simulink model "Copy_of_VTOLTiltrotor"  (R2024a)
settings: configuration reference "VTOLConfiguration" (kept outside this file)
undefined symbols (not defined in the file): airspeed, Battery, BCE12, BCE_Set_init, BMS_Controller_State, C, Cell10_P, Cell11_P, Cell12_P, Cell1_N, Cell1_P, Cell2_P, Cell3_P, Cell4_P, Cell5_P, Cell6_P, Cell7_P, Cell8_P, Cell9_P, Cell_Temperatures, Cell_Voltages, Charging_State, CityMission, control, controlParams, ControlSampleTime, CriticalTiltAngle, currentFactor, CV_Gain, ddx, ddy, ddz, Device_01, DiscIntNeverNeededParam, dx, dy, dz, Earth, env, F, F28379D_ADC_MaxCount, F28379D_ADC_Vmax, FixedWingMission, flightState, Foc_Ki_IxTcpu, Foc_Ki_S, Foc_Kp_I, Foc_Kp_S, fractalcoef, FSState, FWControlParams, HoverMission, I_cc, Ia_offset, Ib_offset, iniRoll, initPitch, iniYaw, IO334, IO334_DAC_Vmax ... (+55)
libraries: slrealtimeethercatlib x109, simulink x81, fl_lib x65, slpidlib x49, mcbcontrolslib x48, nesl_utility x43, speedgoatlib_hdlCoder_IO3xx x31, canmsglib x17, slrealtimeutilitieslib x13, mcbhdlplantlib x13, speedgoatlib_IO611 x12, dspstat3 x12
(part 7 of 20)

== system Copy_of_VTOLTiltrotor/Flight Controller/Autopilot/Tilt Scheduler/Back Transition Scheduler ==
  Tilt Schedule : Inport
  FlightMode : Inport  Port=2
  States : Inport  Port=3
  Add : Sum  Inputs=+-
  Bus Selector : BusSelector  OutputSignals=Vb
  Constant1 : Constant  Value=flightState.BackTransition
  Constant6 : Constant  Value=0
  Equal1 : RelationalOperator  Operator===  OutDataTypeStr=boolean  RndMeth=Simplest  InputSameDT=off
  Saturation : Saturate  UpperLimit=pi/4  LowerLimit=-pi/4
  Selector : Selector  InputPortWidth=3  IndexOptions=Index vector (dialog)  Indices=[1]  OutputSizes=1
  Switch2 : Switch  Threshold=1  SaturateOnIntegerOverflow=off  InputSameDT=off
  Vx Controller : slpidlib/PID Controller  Controller=P  Form=Parallel  TimeDomain=Discrete-time  UseExternalTs=off  SampleTime=0.005  IntegratorMethod=Forward Euler  FilterMethod=Forward Euler  ControllerParametersSource=internal  P=controlParams.P_BACK  I=0  UseKiTs=off  D=0.0379422021775223  UseExternalDerivativeSource=off  N=1.96946409823213  UseFilter=on  TunerSelectOption=Transfer Function Based (PID Tuner App)  InitialConditionSource=internal  InitialConditionForIntegrator=0  InitialConditionForFilter=0  DifferentiatorICPrevScaledInput=0  ExternalReset=none  TrackingMode=off  Kt=1  LimitOutput=off  SatLimitsSource=internal  UpperSaturationLimit=inf  LowerSaturationLimit=-inf  LinearizeAsGain=on  AntiWindupMode=none  Kb=1  LimitIntegrator=off  UpperIntegratorSaturationLimit=inf  LowerIntegratorSaturationLimit=-inf  POutMin=[]  POutMax=[]  IOutMin=[]  IOutMax=[]  DOutMin=[]  DOutMax=[]  NOutMin=[]  NOutMax=[]  SumOutMin=[]  SumOutMax=[]  SaturationOutMin=[]  SaturationOutMax=[]  PParamMin=[]  PParamMax=[]  IParamMin=[]  IParamMax=[]  DParamMin=[]  DParamMax=[]  NParamMin=[]  NParamMax=[]  KbParamMin=[]  KbParamMax=[]  KtParamMin=[]  KtParamMax=[]  KbOutMin=[]  KbOutMax=[]  KtOutMin=[]  KtOutMax=[]  IntegratorOutMin=[]  IntegratorOutMax=[]  FilterOutMin=[]  FilterOutMax=[]  SumI1OutMin=[]  SumI1OutMax=[]  SumI2OutMin=[]  SumI2OutMax=[]  SumI3OutMin=[]  SumI3OutMax=[]  SumI4OutMin=[]  SumI4OutMax=[]  SumDOutMin=[]  SumDOutMax=[]  DifferentiatorOutMin=[]  DifferentiatorOutMax=[]  FilterDiffOutCoefMin=[]  FilterDiffOutCoefMax=[]  ReciprocalOutMin=[]  ReciprocalOutMax=[]  SumDenOutMin=[]  SumDenOutMax=[]  SumNumOutMin=[]  SumNumOutMax=[]  DivideOutMin=[]  DivideOutMax=[]  UdiffTsProdOutMin=[]  UdiffTsProdOutMax=[]  NTsProdOutMin=[]  NTsProdOutMax=[]  UintegralTsProdOutMin=[]  UintegralTsProdOutMax=[]  UngainTsProdOutMin=[]  UngainTsProdOutMax=[]  ClampingZeroOutDataTypeStr=Inherit: Inherit via back propagation  ClampingZeroOutMin=[]  ClampingZeroOutMax=[]  FilterDenConstantOutDataTypeStr=Inherit: Inherit via back propagation  FilterDenConstantOutMin=[]  FilterDenConstantOutMax=[]  PCopyOutDataTypeStr=Inherit: Inherit via back propagation  PCopyOutMin=[]  PCopyOutMax=[]  NCopyOutDataTypeStr=Inherit: Inherit via back propagation  NCopyOutMin=[]  NCopyOutMax=[]  IntegratorContinuousStateAttributes=''  IntegratorStateMustResolveToSignalObject=off  IntegratorRTWStateStorageClass=Auto  FilterContinuousStateAttributes=''  FilterStateMustResolveToSignalObject=off  FilterRTWStateStorageClass=Auto  ParallelPVariant=InternalParameters  IdealPVariant=Disabled  IVariant=Disabled  DVariant=Disabled  IntegratorVariant=Disabled  SatVariant=Disabled  AWVariant=Disabled  PCopyVariant=Disabled  TRVariant=Disabled  FdbkBlocksVariant=Forward  IdealPFdbkVariant=Disabled  SatFdbkVariant=Disabled  DerivativeFilterVariant=Disabled  NVariant=Disabled  NCopyVariant=Disabled_SignalSpec  FilterICVariant=Disabled  IntegratorICVariant=Disabled  ExternalResetVariant=Disabled  TRSumVariant=Passthrough  SumFdbkVariant=Disabled  SumVariant=Passthrough_P  TsampFilterVariant=InternalTs  TsampNgainVariant=Passthrough  TsampIntegralVariant=Disabled_SignalSpec  ExternalSaturationOutDataTypeStr=Inherit: Same as second input  DerivativeSourceVariant=Disabled
  TiltAngle : Outport
  wires:
  States/1 -> Bus Selector/1
  Add/1 -> Vx Controller/1
  Equal1/1 -> Switch2/2
  Bus Selector/1 -> Selector/1  "<Vb>"
  FlightMode/1 -> Equal1/1
  Constant1/1 -> Equal1/2
  Constant6/1 -> Add/1
  Selector/1 -> Add/2
  Vx Controller/1 -> Saturation/1
  Saturation/1 -> Switch2/1
  Tilt Schedule/1 -> Switch2/3
  Switch2/1 -> TiltAngle/1

== system Copy_of_VTOLTiltrotor/Flight Controller/Autopilot/Tilt Scheduler/Forward Transition Scheduler ==
  FlightMode : Inport
  Constant : Constant  Value=pi/2
  Constant2 : Constant  Value=0
  Constant3 : Constant  Value=CriticalTiltAngle
  Constant4 : Constant  Value=flightState.Transition
  Constant5 : Constant  Value=TiltScheduleRate
  Equal : RelationalOperator  Operator===  OutDataTypeStr=boolean  RndMeth=Simplest  InputSameDT=off
  Integrator : Integrator  ExternalReset=either  LimitOutput=on  UpperSaturationLimit=Inf  LowerSaturationLimit=0
  LessThanOrEqual : RelationalOperator  Operator=<=  OutDataTypeStr=boolean  RndMeth=Simplest  InputSameDT=off
  Switch : Switch  Criteria=u2 > Threshold  SaturateOnIntegerOverflow=off  InputSameDT=off
  Switch1 : Switch  Criteria=u2 > Threshold  SaturateOnIntegerOverflow=off  InputSameDT=off
  FlightState : Outport
  Tilt Schedule : Outport  Port=2
  tag scope: ModeFlag=global
  wires:
  FlightMode/1 -> FlightState/1, Equal/2
  [ModeFlag] -> Switch1/2, Integrator/2
  Integrator/1 -> Switch/1, LessThanOrEqual/1
  LessThanOrEqual/1 -> Switch/2
  Equal/1 -> [ModeFlag]
  Constant3/1 -> LessThanOrEqual/2
  Switch1/1 -> Integrator/1
  Constant5/1 -> Switch1/1
  Constant2/1 -> Switch1/3
  Constant4/1 -> Equal/1
  Constant/1 -> Switch/3
  Switch/1 -> Tilt Schedule/1

== system Copy_of_VTOLTiltrotor/Flight Controller/Estimator/Estimation Filter/Airspeed Filter ==
  DiffPress : Inport
  rho : Inport  Port=2
  Constant : Constant  Value=0.5
  Divide : Product  Inputs=*/
  Product : Product
  Sqrt : Sqrt
  airspeed : Outport
  wires:
  Constant/1 -> Product/2
  rho/1 -> Product/1
  Product/1 -> Divide/2
  DiffPress/1 -> Divide/1
  Divide/1 -> Sqrt/1
  Sqrt/1 -> airspeed/1

== system Copy_of_VTOLTiltrotor/Flight Controller/Estimator/Estimation Filter/LLA2Local ==
  LLA : Inport
  Constant1 : Constant  Value=0
  Demux1 : Demux  Outputs=2
  LLA to Flat Earth1 : aerolibtransform2/LLA to Flat Earth  units=Metric (MKS)  ptype=Earth (WGS84)  F=1/298.257223563  R=6378137  refPosPort=off  LL0=[0 0]  psi=0
  Xe : Outport
  wires:
  Constant1/1 -> LLA to Flat Earth1/3
  Demux1/1 -> LLA to Flat Earth1/1
  Demux1/2 -> LLA to Flat Earth1/2
  LLA to Flat Earth1/1 -> Xe/1  "Xe"
  LLA/1 -> Demux1/1

== system Copy_of_VTOLTiltrotor/Flight Controller/Ground Control Station/Get Flight Mission/noQGC ==
  note: uavPathManagerBus type
  No Mission : Constant  Value=struct('mode',0,'position',[0 0 0]','params',[0;0;0;0]);  OutDataTypeStr=Bus: doubleUavPathManager
  Variant Source : VariantSource
  Waypoints : Constant  Value=FixedWingMission  OutDataTypeStr=Bus: doubleUavPathManager  SampleTime=-1
  Waypoints1 : Constant  Value=HoverMission  OutDataTypeStr=Bus: doubleUavPathManager  SampleTime=-1
  Waypoints2 : Constant  Value=TransitionMission  OutDataTypeStr=Bus: doubleUavPathManager  SampleTime=-1
  Waypoints3 : Constant  Value=CityMission  OutDataTypeStr=Bus: doubleUavPathManager  SampleTime=-1
  Mission : Outport
  wires:
  Waypoints/1 -> Variant Source/2
  Waypoints1/1 -> Variant Source/3
  Variant Source/1 -> Mission/1
  Waypoints2/1 -> Variant Source/4
  No Mission/1 -> Variant Source/1
  Waypoints3/1 -> Variant Source/5

== system Copy_of_VTOLTiltrotor/Flight Controller/Guidance Test Bench/ControlType/Guidance Testbench ==
  Global Mission : Inport
  Aircraft States : Inport  Port=2
  Control Rate Transition : Subsystem
  Guidance Logic : Subsystem  VariantControl=guidanceType==1
  HoverCmds : Outport
  FixedWingSP : Outport  Port=2
  AACSP : Outport  Port=3
  ctrlMode : Outport  Port=4
  FlightMode : Outport  Port=5
  wires:
  Aircraft States/1 -> Guidance Logic/1(UAVState)
  Global Mission/1 -> Guidance Logic/2(GCSCommands)
  Guidance Logic/1(HoverGuidance) -> Control Rate Transition/1("1 ")
  Guidance Logic/2(FixedWingSP) -> Control Rate Transition/2(In2)
  Guidance Logic/3(AACSP) -> Control Rate Transition/3(In3)
  Guidance Logic/4(ctrlMode) -> Control Rate Transition/4(In4)
  Guidance Logic/5(FlightMode) -> Control Rate Transition/5(In5)
  Control Rate Transition/1(Out1) -> HoverCmds/1
  Control Rate Transition/2(Out2) -> FixedWingSP/1
  Control Rate Transition/3(Out3) -> AACSP/1
  Control Rate Transition/4(Out4) -> ctrlMode/1
  Control Rate Transition/5(Out5) -> FlightMode/1

== system Copy_of_VTOLTiltrotor/Flight Controller/Guidance Test Bench/ControlType/Manual Control ==
  note: Change these parameters during simulation when using manual testbench mode.
  note: Commanded Altitude (m)
  note: Commanded Y (m)
  note: Fixed Wing Aerodynamics
  note: Commanded X (m)
  note: Fixed Wing
  note: Hover
  note: Flight Mode
  note: Transition
  note: Commanded Course
  note: Commanded Altitude
  note: Commanded Airspeed (m)
  note: Back Transition
  note: Fixed Wing Commands
  note: Hover Commands
  Global Mission : Inport
  Aircraft States : Inport  Port=2
  Command Interface : Subsystem
  Slider1 : SliderBlock  LabelPosition=Hide  ScaleMax=50  TickInterval=5
  Slider2 : SliderBlock  LabelPosition=Hide  ScaleMin=-30  ScaleMax=30  TickInterval=5
  Slider3 : SliderBlock  LabelPosition=Hide  ScaleMin=-30  ScaleMax=30  TickInterval=5
  Slider4 : SliderBlock  LabelPosition=Hide  ScaleMax=3  TickInterval=1
  Slider5 : SliderBlock  LabelPosition=Hide  ScaleMin=-30  ScaleMax=30  TickInterval=5
  Slider6 : SliderBlock  LabelPosition=Hide  ScaleMin=-100  TickInterval=10
  Slider7 : SliderBlock  LabelPosition=Hide  ScaleMin=10  ScaleMax=30  TickInterval=5
  Toggle Switch1 : ToggleSwitchBlock  LabelPosition=Hide
      settings: Values={{'Off', 'On'}, [0 1]}
  HoverCmds : Outport
  FixedWingSP : Outport  Port=2
  AACSP : Outport  Port=3
  ctrlMode : Outport  Port=4
  FlightMode : Outport  Port=5
  wires:
  Global Mission/1 -> Command Interface/1(Global Mission)
  Aircraft States/1 -> Command Interface/2(Aircraft States)
  Command Interface/1(ctrlMode) -> ctrlMode/1
  Command Interface/2(FixedWingSP) -> FixedWingSP/1
  Command Interface/3(AACSP) -> AACSP/1
  Command Interface/4(PositionCmds) -> HoverCmds/1
  Command Interface/5(FlightMode) -> FlightMode/1

== system Copy_of_VTOLTiltrotor/Flight Controller/Guidance Test Bench/Reference Tracking /Fixed Wing Reference ==
  AAC Commands : Inport
  States : Inport  Port=2
  Bus Creator1 : BusCreator  Inputs=2
  Bus Creator2 : BusCreator  Inputs=3
  Bus Selector : BusSelector  OutputSignals=airspeed,Xe,course
  Bus Selector3 : BusSelector  OutputSignals=airspeed,altitude,course
  Gain : Gain  Gain=-1
  Mux1 : Mux  Inputs=3
  Selector : Selector  InputPortWidth=3  IndexOptions=Index vector (dialog)  Indices=3  OutputSizes=1
  To Workspace1 : ToWorkspace  VariableName=FixedWingCmdFdbk  SaveFormat=Structure With Time  SampleTime=-1
  wires:
  Selector/1 -> Gain/1
  Bus Selector3/1 -> Mux1/1  "<airspeed>"
  Bus Selector/1 -> Bus Creator2/1  "<airspeed>"
  Bus Selector3/2 -> Mux1/2  "<altitude>"
  Bus Selector/3 -> Bus Creator2/3  "<course>"
  Mux1/1 -> Bus Creator1/1
  Bus Creator1/1 -> To Workspace1/1
  Bus Selector3/3 -> Mux1/3  "<course>"
  Gain/1 -> Bus Creator2/2  "altitude"
  Bus Creator2/1 -> Bus Creator1/2
  AAC Commands/1 -> Bus Selector3/1
  Bus Selector/2 -> Selector/1  "<Xe>"
  States/1 -> Bus Selector/1

== system Copy_of_VTOLTiltrotor/Flight Controller/Guidance Test Bench/Reference Tracking /Hover Reference ==
  Position Command : Inport
  Position Reference : Inport  Port=2
  Bus Creator : BusCreator  Inputs=2
  Bus Selector1 : BusSelector  OutputSignals=Xe  OutputAsBus=on
  Bus Selector2 : BusSelector  OutputSignals=X,Y,Z
  Mux : Mux  Inputs=3
  To Workspace : ToWorkspace  VariableName=PositionCmdFdbk  SaveFormat=Structure With Time  SampleTime=-1
  wires:
  Position Reference/1 -> Bus Selector1/1
  Bus Selector2/3 -> Mux/3  "<Z>"
  Bus Selector2/1 -> Mux/1  "<X>"
  Bus Selector1/1 -> Bus Creator/2
  Bus Creator/1 -> To Workspace/1
  Bus Selector2/2 -> Mux/2  "<Y>"
  Mux/1 -> Bus Creator/1
  Position Command/1 -> Bus Selector2/1

== system Copy_of_VTOLTiltrotor/Flight Controller/Guidance Test Bench/Reference Tracking /Transition Reference ==
  States : Inport
  Bus Creator : BusCreator  Inputs=4
  Bus Selector4 : BusSelector  OutputSignals=airspeed,RotorParameters.Rotor A,Euler,Xe
  Gain : Gain  Gain=-1
  Selector : Selector  InputPortWidth=3  IndexOptions=Index vector (dialog)  Indices=[2]  OutputSizes=1
  Selector1 : Selector  InputPortWidth=3  IndexOptions=Index vector (dialog)  Indices=[3]  OutputSizes=1
  To Workspace1 : ToWorkspace  VariableName=TransitionFeedback  SaveFormat=Structure With Time  SampleTime=-1
  wires:
  States/1 -> Bus Selector4/1
  Bus Selector4/3 -> Selector/1  "<Euler>"
  Bus Selector4/4 -> Selector1/1  "<Xe>"
  Selector1/1 -> Gain/1
  Bus Selector4/1 -> Bus Creator/1  "<airspeed>"
  Selector/1 -> Bus Creator/3  "pitch"
  Gain/1 -> Bus Creator/4  "altitude"
  Bus Selector4/2 -> Bus Creator/2  "<Rotor A>"
  Bus Creator/1 -> To Workspace1/1

== system Copy_of_VTOLTiltrotor/Motor Control/Controller/Controller_HIL_CAN/CAN Communication 611 ==
  Speed_CMD_rpm : Inport
  Closed_loop : Inport  Port=2
  EnablePWM : Inport  Port=3
  Controller_Parameters : Inport  Port=4
  Bus Selector : BusSelector  OutputSignals=Ia_offset,Ib_offset,Kp_S,Ki_S,Kp_I,Ki_IxTcpu
  "CAN Read " : speedgoatlib_IO611/CAN Read   moduleType=IO611  id=1  channel=1  canType=CAN (HS)  useBusOut=on  HasMulRead=Specify by IDs  MsgIDlist=[1 2]  isEFF=off  LabelInHex=on  enableInput=off  ts=1e-3  initValues=[611 1 0.001 0 1 1 0 1 0 2 2 1 2]
      settings: LibrarySourceBlock=speedgoatlib_CANLIN_OfA2/CAN/CAN Read
  CAN Unpack : canmsglib/CAN Unpack  MsgList=(none)  MsgName=Speed_TI_Out  MsgIDType=Standard (11-bit identifier)  MsgIdentifier=1  MsgLength=8  SignalInfo={ 'Speed_fbk', '0', '32', 'LE', 'single', 'Standard', '0', '1', '0', '-Inf', 'Inf'; 'Pos_fbk', '32', '32', 'LE', 'single', 'Standard', '0', '1', '0', '-Inf', 'Inf' }  IDPort=off  TimestampPort=off  ErrorPort=off  RemotePort=off  LengthPort=off  StatusPort=off  ApplyMinMax=off
      settings: LibrarySourceBlock=canlib/CAN Unpack
  CAN Unpack2 : canmsglib/CAN Unpack  MsgList=(none)  MsgName=Speed_Cmd_fbk  MsgIDType=Standard (11-bit identifier)  MsgIdentifier=2  MsgLength=8  SignalInfo={ 'Speed_Cmd', '0', '32', 'LE', 'single', 'Standard', '0', '1', '0', '-Inf', 'Inf'; 'Spd_pot', '32', '32', 'LE', 'single', 'Standard', '0', '1', '0', '-Inf', 'Inf' }  IDPort=off  TimestampPort=off  ErrorPort=off  RemotePort=off  LengthPort=off  StatusPort=off  ApplyMinMax=off
      settings: LibrarySourceBlock=canlib/CAN Unpack
  "CAN Write " : speedgoatlib_IO611/CAN Write   moduleType=IO611  id=1  channel=1  canType=CAN (HS)  useBusIn=on  numOfMsg=4  enableInput=on  enableStatusPort=off  initValues=[611 1 0.2 0 1 1 0 4 1 1]  ts=Ts_CAN_Tx
      settings: LibrarySourceBlock=speedgoatlib_CANLIN_OfA2/CAN/CAN Write
  "CAN and LIN Setup " : speedgoatlib_IO611/CAN and LIN Setup   moduleInitValues="[611    1    1   -1   -1]"  id=1  moduleType=IO611  pciSlot=-1  canChn1=CAN (HS)  canChn2=Disabled  canChn3=Disabled  canChn4=Disabled  linChn1=Disabled  linChn2=Disabled  canInitStructArray=[]  canTermStructArray=[]  canChn1InitValues="[2   2   1  31   8   2   1   5   2]"  arbBdrChn1=1.0 MBaud  arbManBdrChn1=[2,1,31,8]  fdBdrChn1=5.0 MBaud  fdManBdrChn1=[2,1,5,2]  canChn2InitValues="[1  200    1   31    8    2    1    5    2]"  arbBdrChn2=10 kBaud  arbManBdrChn2=[200,1,31,8]  fdBdrChn2=5.0 MBaud  fdManBdrChn2=[2,1,5,2]  canChn3InitValues="[1   2   1  31   8   2   1   5   2]"  arbBdrChn3=1.0 MBaud  arbManBdrChn3=[2,1,31,8]  fdBdrChn3=5.0 MBaud  fdManBdrChn3=[2,1,5,2]  canChn4InitValues="[1   2   1  31   8   2   1   5   2]"  arbBdrChn4=1.0 MBaud  arbManBdrChn4=[2,1,31,8]  fdBdrChn4=5.0 MBaud  fdManBdrChn4=[2,1,5,2]  bdrLIN1=19200  linChn1InitValues="[1  19200]"  bdrLIN2=19200  linChn2InitValues="[1  19200]"
      settings: SourceProductName=IO611
  CANPack_ManualSignals : canmsglib/CAN Pack  MsgList=(none)  MsgName=Speed_Cmd  MsgIDType=Standard (11-bit identifier)  MsgIdentifier=0  MsgLength=8  Remote=off  ApplyMinMax=off  BusOutput=on  SignalInfo={ 'Speed_Cmd', '0', '32', 'LE', 'single', 'Standard', '0', '1', '0', '-Inf', 'Inf'; 'Closed_loop', '32', '8', 'LE', 'unsigned', 'Standard', '0', '1', '0', '-Inf', 'Inf'; 'EnablePWM', '40', '8', 'LE', 'unsigned', 'Standard', '0', '1', '0', '-Inf', 'Inf'; 'Filler', '48', '16', 'LE', 'signed', 'Standard', '0', '1', '0', '-Inf', 'Inf' }
      settings: DataFormat=manually specified signals
  CANPack_ManualSignals1 : canmsglib/CAN Pack  MsgList=(none)  MsgName=Speed_Parameters  MsgIDType=Standard (11-bit identifier)  MsgIdentifier=31  MsgLength=8  Remote=off  ApplyMinMax=off  BusOutput=on  SignalInfo={ 'Kp_S', '0', '32', 'LE', 'single', 'Standard', '0', '1', '0', '-Inf', 'Inf'; 'Ki_S', '32', '32', 'LE', 'single', 'Standard', '0', '1', '0', '-Inf', 'Inf' }
      settings: DataFormat=manually specified signals
  CANPack_ManualSignals2 : canmsglib/CAN Pack  MsgList=(none)  MsgName=I_Offsets  MsgIDType=Standard (11-bit identifier)  MsgIdentifier=30  MsgLength=8  Remote=off  ApplyMinMax=off  BusOutput=on  SignalInfo={ 'Ia_offset', '0', '32', 'LE', 'single', 'Standard', '0', '1', '0', '-Inf', 'Inf'; 'Ib_offset', '32', '32', 'LE', 'single', 'Standard', '0', '1', '0', '-Inf', 'Inf' }
      settings: DataFormat=manually specified signals
  CANPack_ManualSignals3 : canmsglib/CAN Pack  MsgList=(none)  MsgName=I_Parameters  MsgIDType=Standard (11-bit identifier)  MsgIdentifier=29  MsgLength=8  Remote=off  ApplyMinMax=off  BusOutput=on  SignalInfo={ 'Kp_I', '0', '32', 'LE', 'single', 'Standard', '0', '1', '0', '-Inf', 'Inf'; 'Ki_I', '32', '32', 'LE', 'single', 'Standard', '0', '1', '0', '-Inf', 'Inf' }
      settings: DataFormat=manually specified signals
  Data Type Conversion : DataTypeConversion  OutDataTypeStr=boolean  SaturateOnIntegerOverflow=off  RndMeth=Floor
  Gain{,1..3} (4 alike) : Gain
  Mux : Mux
  Pulse Generator : DiscretePulseGenerator  Period=40  PulseWidth=10  SampleTime=Ts_CAN_Tx/10
  Pulse Generator1 : DiscretePulseGenerator  Period=40  PulseWidth=10  PhaseDelay=10  SampleTime=Ts_CAN_Tx/10
  Pulse Generator2 : DiscretePulseGenerator  Period=40  PulseWidth=10  PhaseDelay=20  SampleTime=Ts_CAN_Tx/10
  Pulse Generator3 : DiscretePulseGenerator  Period=40  PulseWidth=10  PhaseDelay=30  SampleTime=Ts_CAN_Tx/10
  Rate Transition{,1..3,5..9} (9 alike) : RateTransition  Integrity=off  Deterministic=off
  Rate Transition4 : RateTransition  Integrity=off  OutPortSampleTime=Ts_CAN_Tx
  Vector Concatenate : Concatenate  NumInputs=4
  Speed_fbk : Outport
  Pos_fdk : Outport  Port=2
  Speed_Cmd : Outport  Port=3
  Spd_pot : Outport  Port=4
  wires:
  "CAN Read "/2 -> CAN Unpack/1
  CAN Unpack/1 -> Speed_fbk/1
  CAN Unpack/2 -> Pos_fdk/1
  "CAN Read "/3 -> CAN Unpack2/1
  CAN Unpack2/2 -> Spd_pot/1
  CAN Unpack2/1 -> Speed_Cmd/1
  Bus Selector/3 -> Rate Transition6/1  "<Kp_S>"
  Bus Selector/4 -> Rate Transition5/1  "<Ki_S>"
  Bus Selector/2 -> Rate Transition1/1  "<Ib_offset>"
  Bus Selector/1 -> Rate Transition/1  "<Ia_offset>"
  Controller_Parameters/1 -> Bus Selector/1
  Bus Selector/6 -> Rate Transition2/1  "<Ki_IxTcpu>"
  Bus Selector/5 -> Rate Transition3/1  "<Kp_I>"
  CANPack_ManualSignals1/1 -> Vector Concatenate/3  "CAN_Ch1_ID102_Tx"
  CANPack_ManualSignals2/1 -> Vector Concatenate/2  "CAN_Ch1_ID102_Tx"
  Pulse Generator/1 -> Gain3/1
  CANPack_ManualSignals/1 -> Vector Concatenate/1  "CAN_Ch1_ID102_Tx"
  Data Type Conversion/1 -> Rate Transition4/1
  Pulse Generator2/1 -> Gain1/1
  Pulse Generator1/1 -> Gain/1
  Mux/1 -> Data Type Conversion/1
  CANPack_ManualSignals3/1 -> Vector Concatenate/4  "CAN_Ch1_ID102_Tx"
  Pulse Generator3/1 -> Gain2/1
  Rate Transition/1 -> CANPack_ManualSignals2/1
  Rate Transition1/1 -> CANPack_ManualSignals2/2
  Rate Transition6/1 -> CANPack_ManualSignals1/1
  Rate Transition5/1 -> CANPack_ManualSignals1/2
  Rate Transition3/1 -> CANPack_ManualSignals3/1
  Rate Transition2/1 -> CANPack_ManualSignals3/2
  Speed_CMD_rpm/1 -> Rate Transition7/1
  Rate Transition7/1 -> CANPack_ManualSignals/1
  Closed_loop/1 -> Rate Transition8/1
  Rate Transition8/1 -> CANPack_ManualSignals/2
  EnablePWM/1 -> Rate Transition9/1
  Rate Transition9/1 -> CANPack_ManualSignals/3
  Gain3/1 -> Mux/1
  Gain/1 -> Mux/2
  Gain1/1 -> Mux/3
  Gain2/1 -> Mux/4
  Vector Concatenate/1 -> "CAN Write "/2
  Rate Transition4/1 -> "CAN Write "/1

== system Copy_of_VTOLTiltrotor/Motor Control/Controller/Controller_HIL_CAN/Internal PWM configuration1 ==
  Bus Creator1 : BusCreator  Inputs=5
  Not Used Dc : Constant  Value=[0 0 0]  OutDataTypeStr=double
  Not Used Period : Constant  Value=[1 1 1]  OutDataTypeStr=double
  PWM Generation : pwm_cpulib/PWM Generation  f_FPGA=f_FPGA  n_channels=3  sel_scaling=CPU  protection_param=A/B are forced off when A/B are on.  deadband_sec=0  natural_update=At period starts  delay=0  trigger_duration_sec=[1e-6]  trigger_period_start=on  trigger_half_of_the_period=off  trigger_a_on=off  trigger_a_off=off  trigger_b_on=off  trigger_b_off=off  bit_width_pwm_gen=24  invert_a=off  invert_b=on  invert_c=off
      settings: SourceProductName=PWM CPU Library
  bias4 : Constant  Value=0  OutDataTypeStr=boolean  SampleTime=Ts_UI
  bias5 : Constant  Value=0  OutDataTypeStr=boolean  SampleTime=Ts_UI
  bias6 : Constant  OutDataTypeStr=boolean  SampleTime=Ts_UI
  Simu Config : Outport
  wires:
  PWM Generation/2 -> Bus Creator1/3  "PCIe_PWM_Runtime"
  bias6/1 -> Bus Creator1/5  "PCIe_Protocol"
  PWM Generation/1 -> Bus Creator1/2  "PCIe_PWM_Config"
  Bus Creator1/1 -> Simu Config/1
  bias4/1 -> Bus Creator1/1  "PCIe_RC_or_TTL"
  bias5/1 -> Bus Creator1/4  "PCIe_PWM_Enable"
  Not Used Period/1 -> PWM Generation/1
  Not Used Dc/1 -> PWM Generation/2

== system Copy_of_VTOLTiltrotor/Motor Control/Controller/Controller_MIL/F28379D ADC ==
  Iab_IO334V : Inport
  Add Constant : Bias  Bias=Ia_offset  SaturateOnIntegerOverflow=off
  Add Constant1 : Bias  Bias=Ib_offset  SaturateOnIntegerOverflow=off
  Demux : Demux  Outputs=2
  Gain : Gain  Gain=2^12/F28379D_ADC_Vmax
  Ia_ADC : Outport
  Ib_ADC : Outport  Port=2
  wires:
  Iab_IO334V/1 -> Gain/1
  Gain/1 -> Demux/1
  Demux/1 -> Add Constant/1
  Demux/2 -> Add Constant1/1
  Add Constant/1 -> Ia_ADC/1
  Add Constant1/1 -> Ib_ADC/1

== system Copy_of_VTOLTiltrotor/Motor Control/Controller/Controller_MIL/F28379D Firmware ==
  Ia_ADC : Inport
  Ib_ADC : Inport  Port=2
  IaOffset : Inport  Port=3
  IbOffset : Inport  Port=4
  QEP_Position_Count : Inport  Port=5
  QEP_Index_Latch : Inport  Port=6
  SpdCmdRPM : Inport  Port=7
  Kp_S : Inport  Port=8
  Ki_S : Inport  Port=9
  EnClosedLoop : Inport  Port=10
  EnablePWM : Inport  Port=11
  Kp_i : Inport  Port=12
  Ki_ixTcpu : Inport  Port=13
  Controller Algorithm : Subsystem
  Phase_Current_Rescaling : Subsystem
  Speed Conditioning : Subsystem
  ModWave : Outport
  PWM_Enable : Outport  Port=2
  Fbk_CAN : Outport  Port=3
  wires:
  SpdCmdRPM/1 -> Speed Conditioning/1(Spd[rpm])
  Ia_ADC/1 -> Phase_Current_Rescaling/1(Ia_ADC)
  IaOffset/1 -> Phase_Current_Rescaling/3(IaOffset)
  IbOffset/1 -> Phase_Current_Rescaling/4(IbOffset)
  QEP_Position_Count/1 -> Controller Algorithm/2(QEP_Position_Count)
  Controller Algorithm/1(ModWave) -> ModWave/1
  Phase_Current_Rescaling/1(Iab_meas_PU) -> Controller Algorithm/1(Ia_PU)  "Iab_fb_PU"
  Kp_S/1 -> Controller Algorithm/5(Kp_S)
  Controller Algorithm/2(PWM_Enable) -> PWM_Enable/1
  Ki_S/1 -> Controller Algorithm/6(Ki_S)
  QEP_Index_Latch/1 -> Controller Algorithm/3(QEP_Index_Latch)
  Ib_ADC/1 -> Phase_Current_Rescaling/2(Ib_ADC)
  EnClosedLoop/1 -> Controller Algorithm/7(EnClosedLoop)
  EnablePWM/1 -> Controller Algorithm/8(EnablePWM)
  Speed Conditioning/1(Spd[PU]) -> Controller Algorithm/4(SpdCmd)
  Controller Algorithm/3(fbk_CAN) -> Fbk_CAN/1
  Kp_i/1 -> Controller Algorithm/9(Kp_i)
  Ki_ixTcpu/1 -> Controller Algorithm/10(Ki_ixTcpu)

== system Copy_of_VTOLTiltrotor/Motor Control/Controller/Controller_MIL/IO334 DAC ==
  Iab : Inport
  Add : Sum
  Constant : Constant  Value=IO334_iDAC_bias
  Gain : Gain  Gain=IO334_iDAC_gain
  Gain1 : Gain  Gain=2.5/(2^15)
  IO334_DAC_embedded_GAIN : Gain  Gain=2^15/10
  Saturation : Saturate  UpperLimit=IO334_DAC_Vmax  LowerLimit=-IO334_DAC_Vmax
  Iab_IO334DAC : Outport
  wires:
  Iab/1 -> Gain/1
  Gain/1 -> Add/1
  Add/1 -> IO334_DAC_embedded_GAIN/1
  Constant/1 -> Add/2
  IO334_DAC_embedded_GAIN/1 -> Gain1/1
  Gain1/1 -> Saturation/1
  Saturation/1 -> Iab_IO334DAC/1

== system Copy_of_VTOLTiltrotor/Motor Control/Controller1/Controller_MIL/F28379D ADC ==
  Iab_IO334V : Inport
  Add Constant : Bias  Bias=Ia_offset  SaturateOnIntegerOverflow=off
  Add Constant1 : Bias  Bias=Ib_offset  SaturateOnIntegerOverflow=off
  Demux : Demux  Outputs=2
  Gain : Gain  Gain=2^12/F28379D_ADC_Vmax
  Ia_ADC : Outport
  Ib_ADC : Outport  Port=2
  wires:
  Iab_IO334V/1 -> Gain/1
  Gain/1 -> Demux/1
  Demux/1 -> Add Constant/1
  Demux/2 -> Add Constant1/1
  Add Constant/1 -> Ia_ADC/1
  Add Constant1/1 -> Ib_ADC/1

== system Copy_of_VTOLTiltrotor/Motor Control/Controller1/Controller_MIL/F28379D Firmware ==
  Ia_ADC : Inport
  Ib_ADC : Inport  Port=2
  IaOffset : Inport  Port=3
  IbOffset : Inport  Port=4
  QEP_Position_Count : Inport  Port=5
  QEP_Index_Latch : Inport  Port=6
  SpdCmdRPM : Inport  Port=7
  Kp_S : Inport  Port=8
  Ki_S : Inport  Port=9
  EnClosedLoop : Inport  Port=10
  EnablePWM : Inport  Port=11
  Kp_i : Inport  Port=12
  Ki_ixTcpu : Inport  Port=13
  Controller Algorithm : Subsystem
  Phase_Current_Rescaling : Subsystem
  Speed Conditioning : Subsystem
  ModWave : Outport
  PWM_Enable : Outport  Port=2
  Fbk_CAN : Outport  Port=3
  wires:
  SpdCmdRPM/1 -> Speed Conditioning/1(Spd[rpm])
  Ia_ADC/1 -> Phase_Current_Rescaling/1(Ia_ADC)
  IaOffset/1 -> Phase_Current_Rescaling/3(IaOffset)
  IbOffset/1 -> Phase_Current_Rescaling/4(IbOffset)
  QEP_Position_Count/1 -> Controller Algorithm/2(QEP_Position_Count)
  Controller Algorithm/1(ModWave) -> ModWave/1
  Phase_Current_Rescaling/1(Iab_meas_PU) -> Controller Algorithm/1(Ia_PU)  "Iab_fb_PU"
  Kp_S/1 -> Controller Algorithm/5(Kp_S)
  Controller Algorithm/2(PWM_Enable) -> PWM_Enable/1
  Ki_S/1 -> Controller Algorithm/6(Ki_S)
  QEP_Index_Latch/1 -> Controller Algorithm/3(QEP_Index_Latch)
  Ib_ADC/1 -> Phase_Current_Rescaling/2(Ib_ADC)
  EnClosedLoop/1 -> Controller Algorithm/7(EnClosedLoop)
  EnablePWM/1 -> Controller Algorithm/8(EnablePWM)
  Speed Conditioning/1(Spd[PU]) -> Controller Algorithm/4(SpdCmd)
  Controller Algorithm/3(fbk_CAN) -> Fbk_CAN/1
  Kp_i/1 -> Controller Algorithm/9(Kp_i)
  Ki_ixTcpu/1 -> Controller Algorithm/10(Ki_ixTcpu)

== system Copy_of_VTOLTiltrotor/Motor Control/Controller1/Controller_MIL/IO334 DAC ==
  Iab : Inport
  Add : Sum
  Constant : Constant  Value=IO334_iDAC_bias
  Gain : Gain  Gain=IO334_iDAC_gain
  Gain1 : Gain  Gain=2.5/(2^15)
  IO334_DAC_embedded_GAIN : Gain  Gain=2^15/10
  Saturation : Saturate  UpperLimit=IO334_DAC_Vmax  LowerLimit=-IO334_DAC_Vmax
  Iab_IO334DAC : Outport
  wires:
  Iab/1 -> Gain/1
  Gain/1 -> Add/1
  Add/1 -> IO334_DAC_embedded_GAIN/1
  Constant/1 -> Add/2
  IO334_DAC_embedded_GAIN/1 -> Gain1/1
  Gain1/1 -> Saturation/1
  Saturation/1 -> Iab_IO334DAC/1

== system Copy_of_VTOLTiltrotor/Motor Control/Controller2/Controller_MIL/F28379D ADC ==
  Iab_IO334V : Inport
  Add Constant : Bias  Bias=Ia_offset  SaturateOnIntegerOverflow=off
  Add Constant1 : Bias  Bias=Ib_offset  SaturateOnIntegerOverflow=off
  Demux : Demux  Outputs=2
  Gain : Gain  Gain=2^12/F28379D_ADC_Vmax
  Ia_ADC : Outport
  Ib_ADC : Outport  Port=2
  wires:
  Iab_IO334V/1 -> Gain/1
  Gain/1 -> Demux/1
  Demux/1 -> Add Constant/1
  Demux/2 -> Add Constant1/1
  Add Constant/1 -> Ia_ADC/1
  Add Constant1/1 -> Ib_ADC/1

== system Copy_of_VTOLTiltrotor/Motor Control/Controller2/Controller_MIL/F28379D Firmware ==
  Ia_ADC : Inport
  Ib_ADC : Inport  Port=2
  IaOffset : Inport  Port=3
  IbOffset : Inport  Port=4
  QEP_Position_Count : Inport  Port=5
  QEP_Index_Latch : Inport  Port=6
  SpdCmdRPM : Inport  Port=7
  Kp_S : Inport  Port=8
  Ki_S : Inport  Port=9
  EnClosedLoop : Inport  Port=10
  EnablePWM : Inport  Port=11
  Kp_i : Inport  Port=12
  Ki_ixTcpu : Inport  Port=13
  Controller Algorithm : Subsystem
  Phase_Current_Rescaling : Subsystem
  Speed Conditioning : Subsystem
  ModWave : Outport
  PWM_Enable : Outport  Port=2
  Fbk_CAN : Outport  Port=3
  wires:
  SpdCmdRPM/1 -> Speed Conditioning/1(Spd[rpm])
  Ia_ADC/1 -> Phase_Current_Rescaling/1(Ia_ADC)
  IaOffset/1 -> Phase_Current_Rescaling/3(IaOffset)
  IbOffset/1 -> Phase_Current_Rescaling/4(IbOffset)
  QEP_Position_Count/1 -> Controller Algorithm/2(QEP_Position_Count)
  Controller Algorithm/1(ModWave) -> ModWave/1
  Phase_Current_Rescaling/1(Iab_meas_PU) -> Controller Algorithm/1(Ia_PU)  "Iab_fb_PU"
  Kp_S/1 -> Controller Algorithm/5(Kp_S)
  Controller Algorithm/2(PWM_Enable) -> PWM_Enable/1
  Ki_S/1 -> Controller Algorithm/6(Ki_S)
  QEP_Index_Latch/1 -> Controller Algorithm/3(QEP_Index_Latch)
  Ib_ADC/1 -> Phase_Current_Rescaling/2(Ib_ADC)
  EnClosedLoop/1 -> Controller Algorithm/7(EnClosedLoop)
  EnablePWM/1 -> Controller Algorithm/8(EnablePWM)
  Speed Conditioning/1(Spd[PU]) -> Controller Algorithm/4(SpdCmd)
  Controller Algorithm/3(fbk_CAN) -> Fbk_CAN/1
  Kp_i/1 -> Controller Algorithm/9(Kp_i)
  Ki_ixTcpu/1 -> Controller Algorithm/10(Ki_ixTcpu)

== system Copy_of_VTOLTiltrotor/Motor Control/Controller2/Controller_MIL/IO334 DAC ==
  Iab : Inport
  Add : Sum
  Constant : Constant  Value=IO334_iDAC_bias
  Gain : Gain  Gain=IO334_iDAC_gain
  Gain1 : Gain  Gain=2.5/(2^15)
  IO334_DAC_embedded_GAIN : Gain  Gain=2^15/10
  Saturation : Saturate  UpperLimit=IO334_DAC_Vmax  LowerLimit=-IO334_DAC_Vmax
  Iab_IO334DAC : Outport
  wires:
  Iab/1 -> Gain/1
  Gain/1 -> Add/1
  Add/1 -> IO334_DAC_embedded_GAIN/1
  Constant/1 -> Add/2
  IO334_DAC_embedded_GAIN/1 -> Gain1/1
  Gain1/1 -> Saturation/1
  Saturation/1 -> Iab_IO334DAC/1

== system Copy_of_VTOLTiltrotor/Motor Control/Controller3/Controller_MIL/F28379D ADC ==
  Iab_IO334V : Inport
  Add Constant : Bias  Bias=Ia_offset  SaturateOnIntegerOverflow=off
  Add Constant1 : Bias  Bias=Ib_offset  SaturateOnIntegerOverflow=off
  Demux : Demux  Outputs=2
  Gain : Gain  Gain=2^12/F28379D_ADC_Vmax
  Ia_ADC : Outport
  Ib_ADC : Outport  Port=2
  wires:
  Iab_IO334V/1 -> Gain/1
  Gain/1 -> Demux/1
  Demux/1 -> Add Constant/1
  Demux/2 -> Add Constant1/1
  Add Constant/1 -> Ia_ADC/1
  Add Constant1/1 -> Ib_ADC/1

== system Copy_of_VTOLTiltrotor/Motor Control/Controller3/Controller_MIL/F28379D Firmware ==
  Ia_ADC : Inport
  Ib_ADC : Inport  Port=2
  IaOffset : Inport  Port=3
  IbOffset : Inport  Port=4
  QEP_Position_Count : Inport  Port=5
  QEP_Index_Latch : Inport  Port=6
  SpdCmdRPM : Inport  Port=7
  Kp_S : Inport  Port=8
  Ki_S : Inport  Port=9
  EnClosedLoop : Inport  Port=10
  EnablePWM : Inport  Port=11
  Kp_i : Inport  Port=12
  Ki_ixTcpu : Inport  Port=13
  Controller Algorithm : Subsystem
  Phase_Current_Rescaling : Subsystem
  Speed Conditioning : Subsystem
  ModWave : Outport
  PWM_Enable : Outport  Port=2
  Fbk_CAN : Outport  Port=3
  wires:
  SpdCmdRPM/1 -> Speed Conditioning/1(Spd[rpm])
  Ia_ADC/1 -> Phase_Current_Rescaling/1(Ia_ADC)
  IaOffset/1 -> Phase_Current_Rescaling/3(IaOffset)
  IbOffset/1 -> Phase_Current_Rescaling/4(IbOffset)
  QEP_Position_Count/1 -> Controller Algorithm/2(QEP_Position_Count)
  Controller Algorithm/1(ModWave) -> ModWave/1
  Phase_Current_Rescaling/1(Iab_meas_PU) -> Controller Algorithm/1(Ia_PU)  "Iab_fb_PU"
  Kp_S/1 -> Controller Algorithm/5(Kp_S)
  Controller Algorithm/2(PWM_Enable) -> PWM_Enable/1
  Ki_S/1 -> Controller Algorithm/6(Ki_S)
  QEP_Index_Latch/1 -> Controller Algorithm/3(QEP_Index_Latch)
  Ib_ADC/1 -> Phase_Current_Rescaling/2(Ib_ADC)
  EnClosedLoop/1 -> Controller Algorithm/7(EnClosedLoop)
  EnablePWM/1 -> Controller Algorithm/8(EnablePWM)
  Speed Conditioning/1(Spd[PU]) -> Controller Algorithm/4(SpdCmd)
  Controller Algorithm/3(fbk_CAN) -> Fbk_CAN/1
  Kp_i/1 -> Controller Algorithm/9(Kp_i)
  Ki_ixTcpu/1 -> Controller Algorithm/10(Ki_ixTcpu)

== system Copy_of_VTOLTiltrotor/Motor Control/Controller3/Controller_MIL/IO334 DAC ==
  Iab : Inport
  Add : Sum
  Constant : Constant  Value=IO334_iDAC_bias
  Gain : Gain  Gain=IO334_iDAC_gain
  Gain1 : Gain  Gain=2.5/(2^15)
  IO334_DAC_embedded_GAIN : Gain  Gain=2^15/10
  Saturation : Saturate  UpperLimit=IO334_DAC_Vmax  LowerLimit=-IO334_DAC_Vmax
  Iab_IO334DAC : Outport
  wires:
  Iab/1 -> Gain/1
  Gain/1 -> Add/1
  Add/1 -> IO334_DAC_embedded_GAIN/1
  Constant/1 -> Add/2
  IO334_DAC_embedded_GAIN/1 -> Gain1/1
  Gain1/1 -> Saturation/1
  Saturation/1 -> Iab_IO334DAC/1

== system Copy_of_VTOLTiltrotor/Motor Control/Three-Phase PMSM Drive/PMSM and average inverter/Encoder Simulation ==
  Theta_m : Inport
  Add1 : Sum  RndMeth=Simplest
  Data Type Conversion7 : DataTypeConversion  OutDataTypeStr=uint16  RndMeth=Simplest  SaturateOnIntegerOverflow=off
  "Get_PU " : Subsystem
  IndexOffset in PU : Constant  Value=0  OutDataTypeStr=single  SampleTime=-1
  Wrap : Subsystem
  pmsm.QEPSlits*4 : Gain  Gain=Maxon_Mile_Nslits*4  OutDataTypeStr=uint16  RndMeth=Simplest
  QEP_Position_Count : Outport
  wires:
  Add1/1 -> Wrap/1(in)
  Theta_m/1 -> "Get_PU "/1(rad)
  pmsm.QEPSlits*4/1 -> Data Type Conversion7/1  "Theta_e"
  Wrap/1(out) -> pmsm.QEPSlits*4/1  "theta_m(ideal)"
  IndexOffset in PU/1 -> Add1/2
  "Get_PU "/1(PU) -> Add1/1
  Data Type Conversion7/1 -> QEP_Position_Count/1

== system Copy_of_VTOLTiltrotor/Motor Control/Three-Phase PMSM Drive/PMSM and average inverter/Ideal Inverter ==
  V_DC : Inport
  Duty Cycle abc : Inport  Port=2
  Data Type Conversion : DataTypeConversion  OutDataTypeStr=single  SaturateOnIntegerOverflow=off  RndMeth=Floor
  Demux : Demux  Outputs=3
  Mux : Mux  Inputs=3
  Product : Product
  Product1 : Product
  Product2 : Product
  Vabc : Outport
  wires:
  V_DC/1 -> Product2/1, Product1/1, Product/1
  Demux/1 -> Product/2
  Duty Cycle abc/1 -> Data Type Conversion/1
  Mux/1 -> Vabc/1
  Data Type Conversion/1 -> Demux/1
  Demux/2 -> Product1/2
  Demux/3 -> Product2/2
  Product/1 -> Mux/1
  Product1/1 -> Mux/2
  Product2/1 -> Mux/3

== system Copy_of_VTOLTiltrotor/Motor Control/Three-Phase PMSM Drive/PMSM and average inverter/PMSM ==
  Config : Inport
  PhaseVolt abc : Inport  Port=2
  LdTrq / Spd : Inport  Port=3
  Constant : Constant  Value=0  OutDataTypeStr=boolean
  PMSM HDL : mcbhdlplantlib/PMSM HDL  VariantControl=pmsmVariant==pmsmEnum.TorqueInput  Ts=-1
      settings: LibrarySourceBlock=mcbhdllib/Electrical Systems/Motors/PMSM HDL
  Info : Outport
  PhaseCurr : Outport  Port=2
  Torque : Outport  Port=3
  RotorMechSpd : Outport  Port=4
  RotorElecAngle : Outport  Port=5
  wires:
  PMSM HDL/5 -> RotorElecAngle/1
  Config/1 -> PMSM HDL/1
  PMSM HDL/4 -> RotorMechSpd/1
  PMSM HDL/3 -> Torque/1
  PMSM HDL/2 -> PhaseCurr/1
  LdTrq / Spd/1 -> PMSM HDL/3
  PhaseVolt abc/1 -> PMSM HDL/2
  PMSM HDL/1 -> Info/1
  Constant/1 -> PMSM HDL/4

== system Copy_of_VTOLTiltrotor/Motor Control/Three-Phase PMSM Drive/PMSM and average inverter/Runtime to DC ==
  PWM_Runtime : Inport
  Demux : Demux  Outputs=15
  Mux : Mux  Inputs=3
  To Dc A1 : Subsystem
  To Dc A2 : Subsystem
  To Dc A3 : Subsystem
  Duty Cycle abc : Outport
  wires:
  PWM_Runtime/1 -> Demux/1  "PCIe_PWM_Runtime"
  Demux/2 -> To Dc A1/1(A_on)
  Demux/3 -> To Dc A1/2(A_off)
  Demux/7 -> To Dc A2/1(A_on)
  Demux/8 -> To Dc A2/2(A_off)
  Demux/12 -> To Dc A3/1(A_on)
  Demux/13 -> To Dc A3/2(A_off)
  To Dc A1/1(Dc) -> Mux/1
  To Dc A2/1(Dc) -> Mux/2
  To Dc A3/1(Dc) -> Mux/3
  Mux/1 -> Duty Cycle abc/1

== system Copy_of_VTOLTiltrotor/Motor Control/Three-Phase PMSM Drive/PMSM and inverter with switching dynamics/DAC Config ==
  I DAC bias : Constant  Value=IO334_iDAC_bias  OutDataTypeStr=single  SampleTime=Ts_UI
  I DAC gain : Constant  Value=IO334_iDAC_gain  OutDataTypeStr=single  SampleTime=Ts_UI
  Plant_Prequency : Constant  Value=1/ts_FPGA_mdl  SampleTime=Ts_UI
  Sig_frequ : Constant  Value=100000  VectorParams1D=off  SampleTime=Ts_UI
  Subsystem : Subsystem
  I_DAC_gain : Outport
  I_DAC_Current : Outport  Port=2
  DAC_reset : Outport  Port=3
  wires:
  Subsystem/1(DAC_reset) -> DAC_reset/1
  Plant_Prequency/1 -> Subsystem/1(Plant_frequency)
  Sig_frequ/1 -> Subsystem/2(SignalFrequency)
  I DAC gain/1 -> I_DAC_gain/1
  I DAC bias/1 -> I_DAC_Current/1

== system Copy_of_VTOLTiltrotor/Motor Control/Three-Phase PMSM Drive/PMSM and inverter with switching dynamics/Encoder Simulation ==
  Theta_m : Inport
  Add1 : Sum  RndMeth=Simplest
  Data Type Conversion7 : DataTypeConversion  OutDataTypeStr=uint16  RndMeth=Simplest  SaturateOnIntegerOverflow=off
  "Get_PU " : Subsystem
  IndexOffset in PU : Constant  Value=0  OutDataTypeStr=single  SampleTime=-1
  Wrap : Subsystem
  pmsm.QEPSlits*4 : Gain  Gain=Maxon_Mile_Nslits*4  OutDataTypeStr=uint16  RndMeth=Simplest
  QEP_Position_Count : Outport
  wires:
  Add1/1 -> Wrap/1(in)
  Theta_m/1 -> "Get_PU "/1(rad)
  pmsm.QEPSlits*4/1 -> Data Type Conversion7/1  "Theta_e"
  Wrap/1(out) -> pmsm.QEPSlits*4/1  "theta_m(ideal)"
  IndexOffset in PU/1 -> Add1/2
  "Get_PU "/1(PU) -> Add1/1
  Data Type Conversion7/1 -> QEP_Position_Count/1
